simulink model "Tunning_Bioinspired_PID_Esquerdo"  (R2024a)
settings: Solver=ode23  StartTime=0.0  StopTime=100  FixedStep=1  MaxStep=0.1  RelTol=1e-3  AbsTol=1e-6
PostLoadFcn:
  | optsiminit
settings Model: Creator=nikita  LastModifiedBy=mathe
settings SolverCC: AutoScaleAbsTol=off  AlgebraicLoopSolver=TrustRegion
settings DataIOCC: SaveFormat=Array  SignalLoggingSaveFormat=ModelDataLogs  SaveTime=off  ReturnWorkspaceOutputs=off  StateSaveName=x  TimeSaveName=t
settings OptimizationCC: BooleanDataType=off  ExpressionDepthLimit=2147483647  InitFltsAndDblsToZero=on  LifeSpan=inf
settings DebuggingCC: SaveWithParameterizedLinksMsg=none  UnderspecifiedInitializationDetection=Classic  MergeDetectMultiDrivingBlocksExec=none  SignalResolutionControl=TryResolveAllWithWarning  MultiTaskDSMMsg=warning  MultiTaskCondExecSysMsg=none  IntegerOverflowMsg=none  FcnCallInpInsideContextMsg=warning  UnconnectedInputMsg=warning  UnconnectedOutputMsg=warning  UnconnectedLineMsg=warning  StateNameClashWarn=warning  SFUnexpectedBacktrackingDiag=warning  SFNoUnconditionalDefaultTransitionDiag=warning  SFExecutionAtInitializationDiag=none  IntegerSaturationMsg=none  ArithmeticOperatorsInVariantConditions=warning
settings HardwareCC: ProdBitPerPointer=32  ProdBitPerSizeT=32  ProdBitPerPtrDiffT=32  ProdLargestAtomicFloat=None  ProdIntDivRoundTo=Undefined  ProdEndianess=Unspecified  ProdWordSize=32  ProdHWDeviceType=32-bit Generic  TargetUnknown=on
settings ModelReferenceCC: EnableRefExpFcnMdlSchedulingChecks=on  PropagateSignalLabelsOutOfModel=off
settings SFSimCC: SimUseLocalCustomCode=off  CustomCodeUndefinedFunction=UseInterfaceOnly
settings RTWCC: RTWUseLocalCustomCode=off  GPUComputeCapability=3.5
settings CodeAppCC: StateflowObjectComments=on
settings GRTTargetCC: TargetFcnLib=ansi_tfl_tmw.mat  TargetLangStandard=C89/C90 (ANSI)  CombineOutputUpdateFcns=off  GRTInterface=on
settings ConfigComp: CovMetricSettings=dw  CovSaveCumulativeToWorkspaceVar=on  CovSaveSingleToWorkspaceVar=on  CovExternalEMLEnable=off

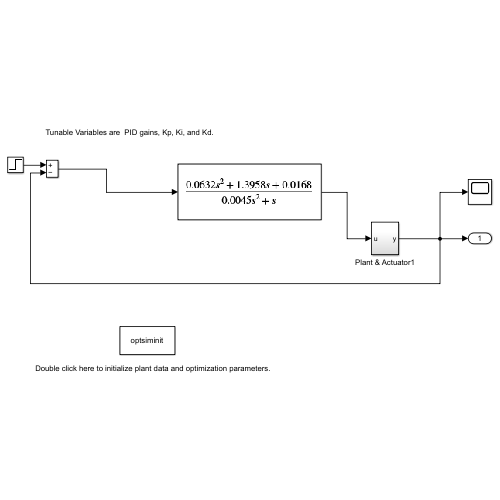
[thumbnail: Simulink's stored preview of the top-level diagram]
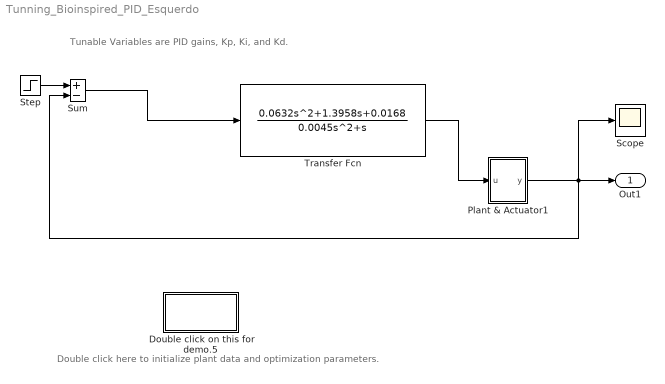
== system Tunning_Bioinspired_PID_Esquerdo ==
  note: Double click here to initialize plant data and optimization parameters.
  note: Tunable Variables are PID gains, Kp, Ki, and Kd.
  Double click on this for demo.5 : Subsystem
      settings: OpenFcn=optsiminit
      mask Display: disp('optsiminit')
  Plant & Actuator1 : Subsystem
  Scope : Scope
  Step : Step  Time=0  After=200  SampleTime=0
  Sum : Sum  Inputs=+-  InputSameDT=on  SaturateOnIntegerOverflow=on  OutDataTypeStr=Inherit: Same as first input
  Transfer Fcn : TransferFcn  Numerator=[0.0632 1.3958 0.0168]  Denominator=[0.0045 1 0]
  Out1 : Outport  VectorParamsAs1DForOutWhenUnconnected=off
  wires:
  Sum/1 -> Transfer Fcn/1
  Step/1 -> Sum/1
  Transfer Fcn/1 -> Plant & Actuator1/1("u ")
  Plant & Actuator1/1(y) -> Sum/2, Out1/1, Scope/1

== system Tunning_Bioinspired_PID_Esquerdo/Double click on this for demo.5 ==

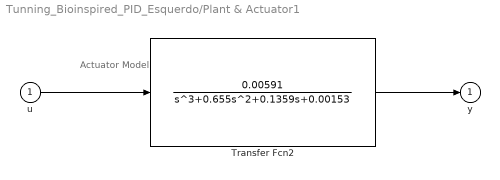
== system Tunning_Bioinspired_PID_Esquerdo/Plant & Actuator1 ==
  note: Actuator Model
  "u " : Inport
  Transfer Fcn2 : TransferFcn  Numerator=[0.00591]  Denominator=[1 0.655 0.1359 0.00153]
  y : Outport  InitialOutput=0  VectorParamsAs1DForOutWhenUnconnected=off
  wires:
  Transfer Fcn2/1 -> y/1
  "u "/1 -> Transfer Fcn2/1
